simulink model "PlDLab3"  (R2025b)
settings: Solver=VariableStepAuto  StartTime=0.0  StopTime=10  RelTol=1e-3
values from neighbouring files (symbols this model uses):
  Beq = B_eq_est    [LAB3_PID.m]
  Jeq = mot.J + mld.Jh / (gbox.N^2)    [LAB3_PID.m]
  Kd = Kp * Td    [LAB3_PID.m]
  Ki = Kp / Ti    [LAB3_PID.m]
  Kp = mag_pid * cos(phi_pid_rad)    [LAB3_PID.m]
  Kw = 1/Tw    (= 5.88235294118)    [LAB3_PID.m]
  Req = mot.R + sens.curr.Rs    [LAB3_PID.m]
  Tl = 1/(10*w_gc)    [LAB3_PID.m]
  Ts = 0.001    [LAB3_PID.m]
undefined symbols (not defined in the file or in its folder): daq, drv, gbox, mld, mot, rads2rpm, sens
settings Model: Creator=super  LastModifiedBy=super

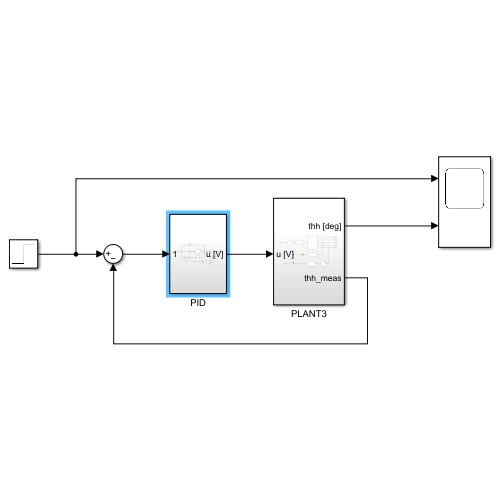
[thumbnail: Simulink's stored preview of the top-level diagram]
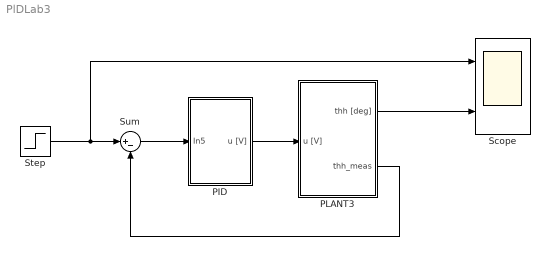
== system PlDLab3 ==
  PID : Subsystem
  PLANT3 : Subsystem
  Scope : Scope  NumInputPorts=2
      settings: ActiveDisplayYMinimum=-29.9670941944892  ActiveDisplayYMaximum=269.28810511223531
  Step : Step  After=120  SampleTime=0
  Sum : Sum  Inputs=|+-
  wires:
  PID/1(u [V]) -> PLANT3/1(u [V])
  PLANT3/1(thh [deg]) -> Scope/2
  Sum/1 -> PID/1(In5)
  Step/1 -> Scope/1, Sum/1
  PLANT3/2(thh_meas) -> Sum/2

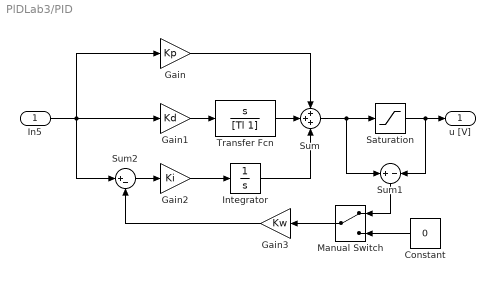
== system PlDLab3/PID ==
  In5 : Inport
  Constant : Constant  Value=0
  Gain : Gain  Gain=Kp
  Gain1 : Gain  Gain=Kd
  Gain2 : Gain  Gain=Ki
  Gain3 : Gain  Gain=Kw
  Integrator : Integrator
  Manual Switch : ManualSwitch
  Saturation : Saturate  UpperLimit=10  LowerLimit=-10
  Sum : Sum  Inputs=+++
  Sum1 : Sum  Inputs=+-
  Sum2 : Sum  Inputs=|+-
  Transfer Fcn : TransferFcn  Numerator=[1 0]  Denominator=[Tl 1]
  u [V] : Outport
  wires:
  Integrator/1 -> Sum/3
  Gain1/1 -> Transfer Fcn/1
  Gain/1 -> Sum/1
  Transfer Fcn/1 -> Sum/2
  Gain2/1 -> Integrator/1
  In5/1 -> Sum2/1, Gain/1, Gain1/1
  Gain3/1 -> Sum2/2
  Sum/1 -> Saturation/1, Sum1/1
  Sum1/1 -> Manual Switch/1
  Saturation/1 -> Sum1/2, u [V]/1
  Sum2/1 -> Gain2/1
  Manual Switch/1 -> Gain3/1
  Constant/1 -> Manual Switch/2

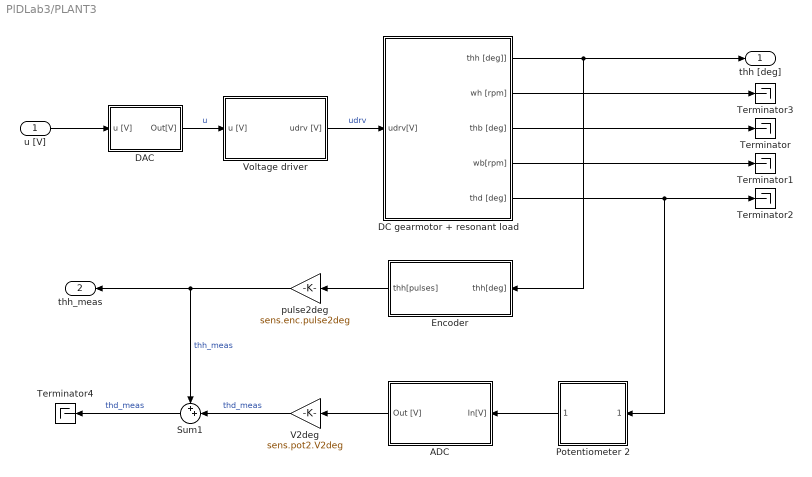
== system PlDLab3/PLANT3 ==
  u [V] : Inport
  ADC : Subsystem
  DAC : Subsystem  TreatAsAtomicUnit=on
  DC gearmotor + resonant load : Subsystem
  Encoder : Subsystem  TreatAsAtomicUnit=on
  Potentiometer 2 : Subsystem
  Sum1 : Sum  Inputs=++|
  Terminator{,1..4} (5 alike) : Terminator
  V2deg : Gain  Gain=sens.pot2.V2deg
  Voltage driver : Subsystem
  pulse2deg : Gain  Gain=sens.enc.pulse2deg
  thh [deg] : Outport
  thh_meas : Outport  Port=2
  wires:
  Encoder/1(thh[pulses]) -> pulse2deg/1
  u [V]/1 -> DAC/1(u [V])
  DC gearmotor + resonant load/1(thh [deg]]) -> Encoder/1(thh[deg]), thh [deg]/1
  DAC/1(Out[V]) -> Voltage driver/1(u [V])  "u"
  Voltage driver/1(udrv [V]) -> DC gearmotor + resonant load/1(udrv[V])  "udrv"
  DC gearmotor + resonant load/3(thb [deg]) -> Terminator/1
  DC gearmotor + resonant load/4(wb[rpm]) -> Terminator1/1
  DC gearmotor + resonant load/5(thd [deg]) -> Terminator2/1, Potentiometer 2/1(thd [deg])
  DC gearmotor + resonant load/2(wh [rpm]) -> Terminator3/1
  Potentiometer 2/1(Out [V]) -> ADC/1(In[V])
  ADC/1(Out [V]) -> V2deg/1
  V2deg/1 -> Sum1/2  "thd_meas"
  pulse2deg/1 -> thh_meas/1, Sum1/1  "thh_meas"
  Sum1/1 -> Terminator4/1  "thd_meas"

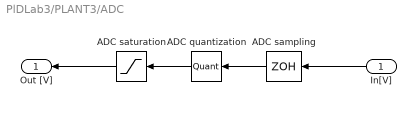
== system PlDLab3/PLANT3/ADC ==
  In[V] : Inport
  " ADC saturation" : Saturate  UpperLimit=daq.adc.fs  LowerLimit=-daq.adc.fs
  ADC quantization : Quantizer  QuantizationInterval=daq.adc.q
  ADC sampling : ZeroOrderHold  SampleTime=Ts
  Out [V] : Outport
  wires:
  ADC sampling/1 -> ADC quantization/1
  ADC quantization/1 -> " ADC saturation"/1
  In[V]/1 -> ADC sampling/1
  " ADC saturation"/1 -> Out [V]/1

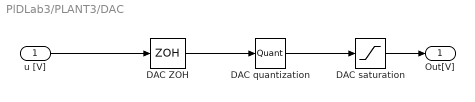
== system PlDLab3/PLANT3/DAC ==
  u [V] : Inport
  "DAC ZOH " : ZeroOrderHold  SampleTime="Ts  %daq.dac.Ts"
  DAC quantization : Quantizer  QuantizationInterval=daq.dac.q
  DAC saturation : Saturate  UpperLimit=daq.dac.fs  LowerLimit=-daq.dac.fs
  Out[V] : Outport
  wires:
  DAC quantization/1 -> DAC saturation/1
  u [V]/1 -> "DAC ZOH "/1
  "DAC ZOH "/1 -> DAC quantization/1
  DAC saturation/1 -> Out[V]/1

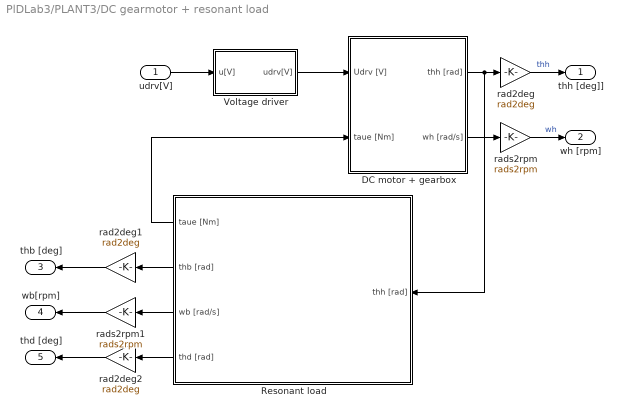
== system PlDLab3/PLANT3/DC gearmotor + resonant load ==
  udrv[V] : Inport
  DC motor + gearbox : Subsystem
  Resonant load : Subsystem
  Voltage driver : Subsystem  TreatAsAtomicUnit=on
  rad2deg : Gain  Gain=rad2deg
  rad2deg1 : Gain  Gain=rad2deg
  rad2deg2 : Gain  Gain=rad2deg
  rads2rpm : Gain  Gain=rads2rpm
  rads2rpm1 : Gain  Gain=rads2rpm
  thh [deg]] : Outport
  wh [rpm] : Outport  Port=2
  thb [deg] : Outport  Port=3
  wb[rpm] : Outport  Port=4
  thd [deg] : Outport  Port=5
  wires:
  Voltage driver/1(udrv[V]) -> DC motor + gearbox/1(Udrv [V])
  udrv[V]/1 -> Voltage driver/1(u[V])
  DC motor + gearbox/1(thh [rad]) -> Resonant load/1(thh [rad]), rad2deg/1
  DC motor + gearbox/2(wh [rad/s]) -> rads2rpm/1
  rad2deg/1 -> thh [deg]]/1  "thh"
  rads2rpm/1 -> wh [rpm]/1  "wh"
  Resonant load/2(thb [rad]) -> rad2deg1/1
  Resonant load/3(wb [rad/s]) -> rads2rpm1/1
  Resonant load/1(taue [Nm]) -> DC motor + gearbox/2(taue [Nm])
  Resonant load/4(thd [rad]) -> rad2deg2/1
  rad2deg1/1 -> thb [deg]/1
  rads2rpm1/1 -> wb[rpm]/1
  rad2deg2/1 -> thd [deg]/1

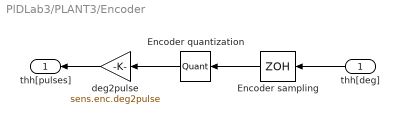
== system PlDLab3/PLANT3/Encoder ==
  thh[deg] : Inport
  Encoder sampling : ZeroOrderHold  SampleTime=Ts%daq.dac.Ts
  Encoder quantization : Quantizer  QuantizationInterval=sens.enc.pulse2deg
  deg2pulse : Gain  Gain=sens.enc.deg2pulse
  thh[pulses] : Outport
  wires:
  Encoder quantization/1 -> deg2pulse/1
  thh[deg]/1 -> Encoder sampling/1
  Encoder sampling/1 -> Encoder quantization/1
  deg2pulse/1 -> thh[pulses]/1

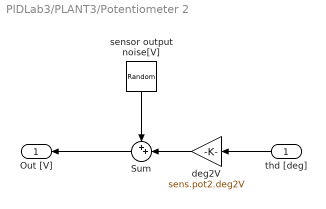
== system PlDLab3/PLANT3/Potentiometer 2 ==
  thd [deg] : Inport
  Sum : Sum  Inputs=++|
  deg2V : Gain  Gain=sens.pot2.deg2V
  sensor output noise[V] : RandomNumber  Variance=3.5e-7  SampleTime=Ts
  Out [V] : Outport
  wires:
  sensor output noise[V]/1 -> Sum/1
  thd [deg]/1 -> deg2V/1
  deg2V/1 -> Sum/2
  Sum/1 -> Out [V]/1

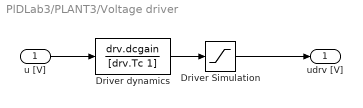
== system PlDLab3/PLANT3/Voltage driver ==
  u [V] : Inport
  Driver Simulation : Saturate
  Driver dynamics : TransferFcn  Numerator=drv.dcgain  Denominator=[drv.Tc 1]
  udrv [V] : Outport
  wires:
  u [V]/1 -> Driver dynamics/1
  Driver Simulation/1 -> udrv [V]/1
  Driver dynamics/1 -> Driver Simulation/1

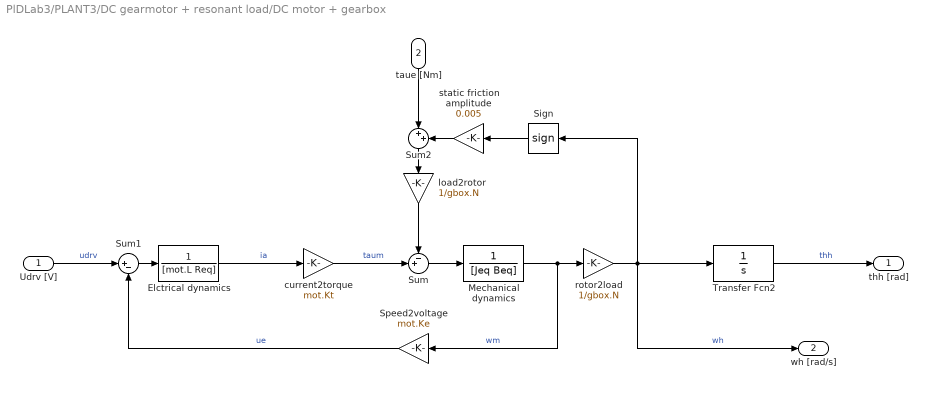
== system PlDLab3/PLANT3/DC gearmotor + resonant load/DC motor + gearbox ==
  Udrv [V] : Inport
  taue [Nm] : Inport  Port=2
  Elctrical dynamics : TransferFcn  Denominator=[mot.L Req]
  Mechanical dynamics : TransferFcn  Denominator=[Jeq Beq]
  Sign : Signum  ZeroCross=off
  Speed2voltage : Gain  Gain=mot.Ke
  Sum : Sum  Inputs=-+|
  Sum1 : Sum  Inputs=|+-
  Sum2 : Sum  Inputs=|++
  Transfer Fcn2 : TransferFcn  Denominator=[1 0]
  current2torque : Gain  Gain=mot.Kt
  load2rotor : Gain  Gain=1/gbox.N
  rotor2load : Gain  Gain=1/gbox.N
  static friction amplitude : Gain  Gain=0.005
  thh [rad] : Outport
  wh [rad/s] : Outport  Port=2
  wires:
  Sign/1 -> static friction amplitude/1
  rotor2load/1 -> wh [rad/s]/1, Sign/1, Transfer Fcn2/1  "wh"
  Sum/1 -> Mechanical dynamics/1
  Udrv [V]/1 -> Sum1/1  "udrv"
  static friction amplitude/1 -> Sum2/2
  load2rotor/1 -> Sum/1
  current2torque/1 -> Sum/2  "taum"
  Speed2voltage/1 -> Sum1/2  "ue"
  Mechanical dynamics/1 -> Speed2voltage/1, rotor2load/1  "wm"
  Elctrical dynamics/1 -> current2torque/1  "ia"
  Sum1/1 -> Elctrical dynamics/1
  Transfer Fcn2/1 -> thh [rad]/1  "thh"
  Sum2/1 -> load2rotor/1
  taue [Nm]/1 -> Sum2/1

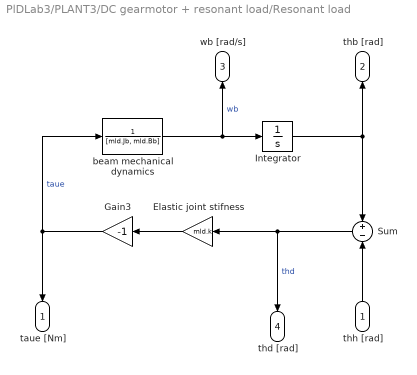
== system PlDLab3/PLANT3/DC gearmotor + resonant load/Resonant load ==
  thh [rad] : Inport
  Elastic joint stifness : Gain  Gain=mld.k
  Gain3 : Gain  Gain=-1
  Integrator : Integrator
  Sum : Sum  Inputs=+-
  beam mechanical dynamics : TransferFcn  Denominator=[mld.Jb, mld.Bb]
  taue [Nm] : Outport
  thb [rad] : Outport  Port=2
  wb [rad/s] : Outport  Port=3
  thd [rad] : Outport  Port=4
  wires:
  beam mechanical dynamics/1 -> wb [rad/s]/1, Integrator/1  "wb"
  Sum/1 -> thd [rad]/1, Elastic joint stifness/1  "thd"
  thh [rad]/1 -> Sum/2
  Integrator/1 -> thb [rad]/1, Sum/1
  Gain3/1 -> beam mechanical dynamics/1, taue [Nm]/1  "taue"
  Elastic joint stifness/1 -> Gain3/1

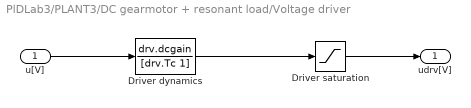
== system PlDLab3/PLANT3/DC gearmotor + resonant load/Voltage driver ==
  u[V] : Inport
  Driver dynamics : TransferFcn  Numerator=drv.dcgain  Denominator=[drv.Tc 1]
  Driver saturation : Saturate  UpperLimit=drv.outmax  LowerLimit=-drv.outmax
  udrv[V] : Outport
  wires:
  Driver dynamics/1 -> Driver saturation/1
  u[V]/1 -> Driver dynamics/1
  Driver saturation/1 -> udrv[V]/1
